simulink model "TwoArea_fromWorkspace_MaxRamp"  (R2017b)
settings: Solver=VariableStepAuto  StartTime=0.0  StopTime=100  RelTol=1e-3  EnableMultiTasking=on
values from neighbouring files (symbols this model uses):
  D = [1e-2 1e-2]    [TwoArea_fromWorkspace2.m]    (also in TwoArea_fromWorkspaceold.m)
  H1 = xvals(xindex)    [TwoArea_fromWorkspace2.m]    (also in TwoArea_fromWorkspaceold.m = 133.22240649)
  H2 = yvals(yindex)    [TwoArea_fromWorkspace2.m]    (also in TwoArea_fromWorkspaceold.m = 2000)
  P_D = 35e3*[1/2 1/2]    [TwoArea_fromWorkspace2.m]    (also in TwoArea_fromWorkspaceold.m = 35e3*[3/4 1/4])
  P_loss = 1.8e3    (= 1800)    [TwoArea_fromWorkspace2.m]    (also in TwoArea_fromWorkspaceold.m)
  PFR1 = PFR1vals(PFR1index)    [TwoArea_fromWorkspace2.m]    (also in TwoArea_fromWorkspaceold.m = 4000)
  PFR2 = PFR2vals(PFR2index)    [TwoArea_fromWorkspace2.m]    (also in TwoArea_fromWorkspaceold.m = 3000)
  Td = 10    [TwoArea_fromWorkspace2.m]    (also in TwoArea_fromWorkspaceold.m)
  V = 345    [TwoArea_fromWorkspace2.m]    (also in TwoArea_fromWorkspaceold.m)
  X = 25    [TwoArea_fromWorkspace2.m]    (also in TwoArea_fromWorkspaceold.m)
libraries: simulink x2
settings Model: Creator=lb2916  LastModifiedBy=keerthanenravichandran
settings OptimizationCC: LifeSpan=inf
settings DebuggingCC: SFUnexpectedBacktrackingDiag=warning  SFNoUnconditionalDefaultTransitionDiag=warning  SFExecutionAtInitializationDiag=none
settings CodeAppCC: StateflowObjectComments=on
settings GRTTargetCC: TargetLangStandard=C89/C90 (ANSI)  GeneratePreprocessorConditionals=Disable all
settings ConfigComp: CovMetricSettings=dw  CovHtmlReporting=on  CovSaveCumulativeToWorkspaceVar=on  CovSaveSingleToWorkspaceVar=on  CovExternalEMLEnable=off

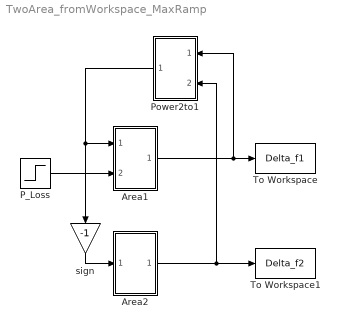
== system TwoArea_fromWorkspace_MaxRamp ==
  Area1 : Subsystem
  Area2 : Subsystem
  P_Loss : Step  Time=1000  Before=P_loss  After=P_loss  SampleTime=0
  Power2to1 : Subsystem
  To Workspace : ToWorkspace  VariableName=Delta_f1  SaveFormat=Timeseries  SampleTime=-1
  To Workspace1 : ToWorkspace  VariableName=Delta_f2  SaveFormat=Timeseries  SampleTime=-1
  sign : Gain  Gain=-1
  wires:
  Area1/1(Out1) -> To Workspace/1, Power2to1/1(In1)
  P_Loss/1 -> Area1/2(In2)
  Area2/1(Out1) -> Power2to1/2(In2), To Workspace1/1
  Power2to1/1(Out1) -> Area1/1(In1), sign/1
  sign/1 -> Area2/1(In1)

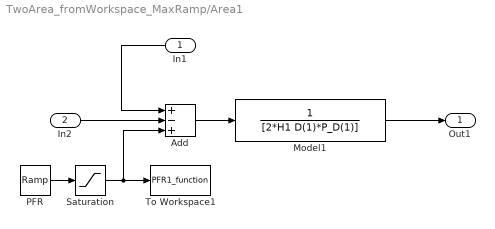
== system TwoArea_fromWorkspace_MaxRamp/Area1 ==
  In1 : Inport
  In2 : Inport  Port=2
  Add : Sum  Inputs=+-+
  Model1 : TransferFcn  Denominator=[2*H1 D(1)*P_D(1)]
  PFR : simulink/Sources/Ramp  slope=PFR1/Td  start=0  X0=0
  Saturation : Saturate  UpperLimit=PFR1  LowerLimit=0
  To Workspace1 : ToWorkspace  VariableName=PFR1_function  SaveFormat=Timeseries  SampleTime=-1
  Out1 : Outport
  wires:
  In2/1 -> Add/2
  Model1/1 -> Out1/1
  Add/1 -> Model1/1
  In1/1 -> Add/1
  Saturation/1 -> Add/3, To Workspace1/1
  PFR/1 -> Saturation/1

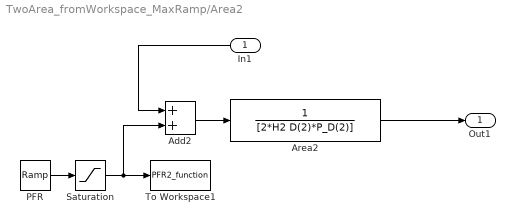
== system TwoArea_fromWorkspace_MaxRamp/Area2 ==
  In1 : Inport
  Add2 : Sum
  Area2 : TransferFcn  Denominator=[2*H2 D(2)*P_D(2)]
  PFR : simulink/Sources/Ramp  slope=PFR2/Td  start=0  X0=0
  Saturation : Saturate  UpperLimit=PFR2  LowerLimit=0
  To Workspace1 : ToWorkspace  VariableName=PFR2_function  SaveFormat=Timeseries  SampleTime=-1
  Out1 : Outport
  wires:
  Area2/1 -> Out1/1
  Add2/1 -> Area2/1
  In1/1 -> Add2/1
  Saturation/1 -> Add2/2, To Workspace1/1
  PFR/1 -> Saturation/1

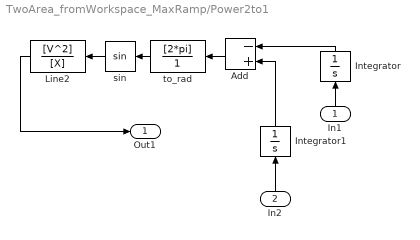
== system TwoArea_fromWorkspace_MaxRamp/Power2to1 ==
  In1 : Inport
  In2 : Inport  Port=2
  Add : Sum  Inputs=-+
  Integrator : Integrator
  Integrator1 : Integrator
  Line2 : TransferFcn  Numerator=[V^2]  Denominator=[X]
  sin : Trigonometry
  to_rad : TransferFcn  Numerator=[2*pi]  Denominator=[1]
  Out1 : Outport
  wires:
  Line2/1 -> Out1/1
  Add/1 -> to_rad/1
  to_rad/1 -> sin/1
  sin/1 -> Line2/1
  In1/1 -> Integrator/1
  Integrator/1 -> Add/1
  In2/1 -> Integrator1/1
  Integrator1/1 -> Add/2
